simulink model "moving_avg_TB"  (R2024a)
settings: Solver=VariableStepAuto  StartTime=0.0  StopTime=2000  RelTol=1e-3
PreLoadFcn:
  | N = 100;
InitFcn:
  | N = 100;
undefined symbols (not defined in the file or in its folder): Ts
libraries: dspbuff3 x1, simulink x1, dspstat3 x1, dspsrcs4 x1
settings Model: Creator=kschutz  LastModifiedBy=kschutz

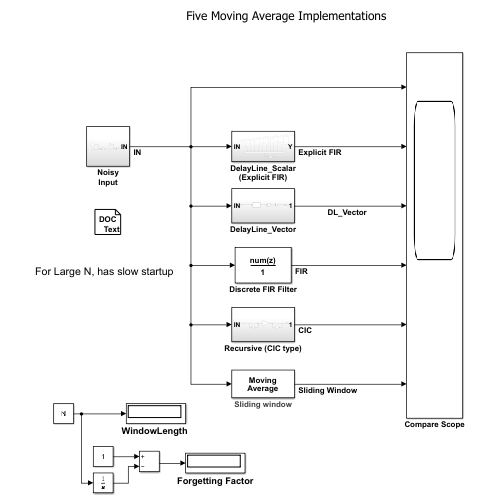
[thumbnail: Simulink's stored preview of the top-level diagram]
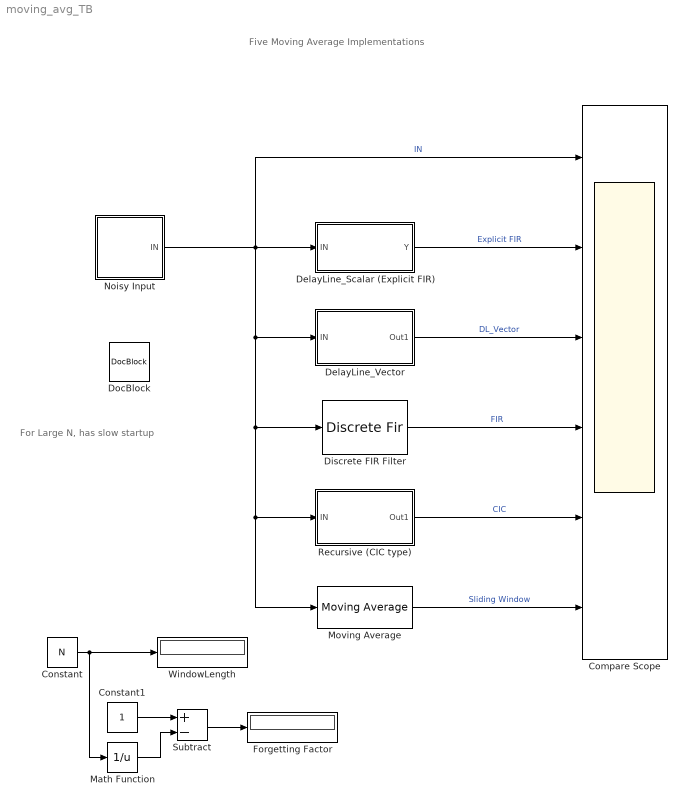
== system moving_avg_TB ==
  note: For Large N, has slow startup
  note: Five Moving Average Implementations
  Compare Scope : Scope  NumInputPorts=6
  Constant : Constant  Value=N
  Constant1 : Constant
  DelayLine_Scalar (Explicit FIR) : Subsystem
  DelayLine_Vector : Subsystem
  Discrete FIR Filter : DiscreteFir  Coefficients=ones(1,N)/N
  DocBlock : simulink/Model-Wide Utilities/DocBlock  DocumentType=Text
      content=|
      | The CIC implementation is the most efficient from a resources perspective,
      | 1 multiplier and two adders. If N is a power of 2, then no multipliers are
      | necessary, just shift logic instead.
  Forgetting Factor : Display
  Math Function : Math  Operator=reciprocal
  Moving Average : dspstat3/Moving Average  Method=Sliding window  ForgettingFactorPort=off  SpecifyWindowLength=on  WindowLength=N  OverlapLength=N-1  AllowArbitraryInputLength=off  ForgettingFactor=1  SimulateUsing=Interpreted execution
      settings: AttributesFormatString=%<Method>
  Noisy Input : Subsystem
  Recursive (CIC type) : Subsystem
  Subtract : Sum  Inputs=+-
  "WindowLength " : Display
  wires:
  Noisy Input/1(IN) -> Compare Scope/1, Moving Average/1, Recursive (CIC type)/1(IN), Discrete FIR Filter/1, DelayLine_Vector/1(IN), DelayLine_Scalar (Explicit FIR)/1(IN)  "IN"
  DelayLine_Scalar (Explicit FIR)/1(Y) -> Compare Scope/2  "Explicit FIR"
  DelayLine_Vector/1(Out1) -> Compare Scope/3  "DL_Vector"
  Discrete FIR Filter/1 -> Compare Scope/4  "FIR"
  Recursive (CIC type)/1(Out1) -> Compare Scope/5  "CIC"
  Moving Average/1 -> Compare Scope/6  "Sliding Window"
  Constant/1 -> "WindowLength "/1, Math Function/1
  Subtract/1 -> Forgetting Factor/1
  Constant1/1 -> Subtract/1
  Math Function/1 -> Subtract/2

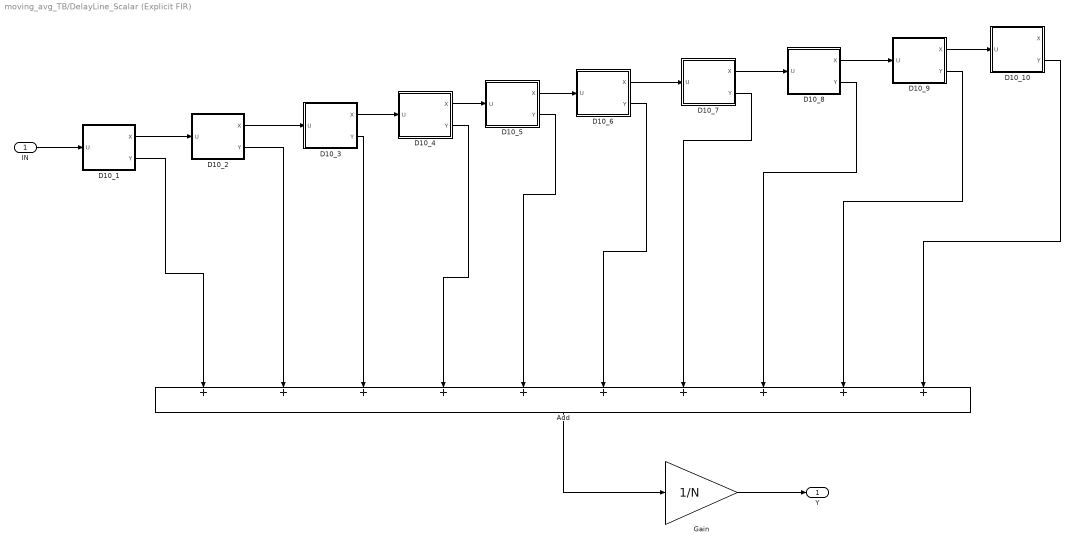
== system moving_avg_TB/DelayLine_Scalar (Explicit FIR) ==
  IN : Inport
  Add : Sum  Inputs=++++++++++
  D10_1 : Subsystem
  D10_10 : Subsystem
  D10_2 : Subsystem
  D10_3 : Subsystem
  D10_4 : Subsystem
  D10_5 : Subsystem
  D10_6 : Subsystem
  D10_7 : Subsystem
  D10_8 : Subsystem
  D10_9 : Subsystem
  Gain : Gain  Gain=1/N
  Y : Outport
  wires:
  IN/1 -> D10_1/1(U)
  D10_1/1(X) -> D10_2/1(U)
  D10_2/1(X) -> D10_3/1(U)
  D10_3/1(X) -> D10_4/1(U)
  D10_4/1(X) -> D10_5/1(U)
  D10_5/1(X) -> D10_6/1(U)
  D10_6/1(X) -> D10_7/1(U)
  D10_7/1(X) -> D10_8/1(U)
  D10_8/1(X) -> D10_9/1(U)
  D10_9/1(X) -> D10_10/1(U)
  D10_1/2(Y) -> Add/1
  Add/1 -> Gain/1
  Gain/1 -> Y/1
  D10_2/2(Y) -> Add/2
  D10_3/2(Y) -> Add/3
  D10_4/2(Y) -> Add/4
  D10_5/2(Y) -> Add/5
  D10_6/2(Y) -> Add/6
  D10_7/2(Y) -> Add/7
  D10_8/2(Y) -> Add/8
  D10_9/2(Y) -> Add/9
  D10_10/2(Y) -> Add/10

== system moving_avg_TB/DelayLine_Vector ==
  IN : Inport
  Delay Line : dspbuff3/Delay Line  siz=N  ic=0  directfeed=on  enable_output=off  hold_output=off  OutputFrames=off
  Gain : Gain  Gain=1/N
  Sum of Elements : Sum  Inputs=+
  Out1 : Outport
  wires:
  Gain/1 -> Out1/1
  Sum of Elements/1 -> Gain/1
  Delay Line/1 -> Sum of Elements/1
  IN/1 -> Delay Line/1

== system moving_avg_TB/Noisy Input ==
  Add : Sum
  Add1 : Sum
  Constant : Constant  SampleTime=1
  Random Source : dspsrcs4/Random Source  SrcType=Gaussian  MinVal=0  MaxVal=1  MeanVal=0  VarVal=.2  RepMode=Specify seed  rawSeed=123  IsInherit=off  SampTime=1  SampFrame=1  OutComplex=Real  DataType=double  SimulateUsing=Interpreted execution
  Step : Step  Time=500  SampleTime=0
  IN : Outport  VectorParamsAs1DForOutWhenUnconnected=off
  wires:
  Constant/1 -> Add1/2
  Random Source/1 -> Add1/1
  Add/1 -> IN/1
  Add1/1 -> Add/2
  Step/1 -> Add/1

== system moving_avg_TB/Recursive (CIC type) ==
  IN : Inport
  Delay : Delay  DelayLength=N
  Delay1 : Delay  DelayLength=1  InputProcessing=Columns as channels (frame based)
  Gain : Gain  Gain=1/N
  Sum : Sum  Inputs=|+-
  Sum1 : Sum  Inputs=|++
  Zero-Order Hold : ZeroOrderHold  Commented=through  SampleTime=Ts
  Out1 : Outport
  wires:
  Sum/1 -> Gain/1
  Sum1/1 -> Out1/1, Delay1/1
  Gain/1 -> Sum1/1
  Delay/1 -> Sum/2
  IN/1 -> Zero-Order Hold/1
  Delay1/1 -> Sum1/2
  Zero-Order Hold/1 -> Delay/1, Sum/1

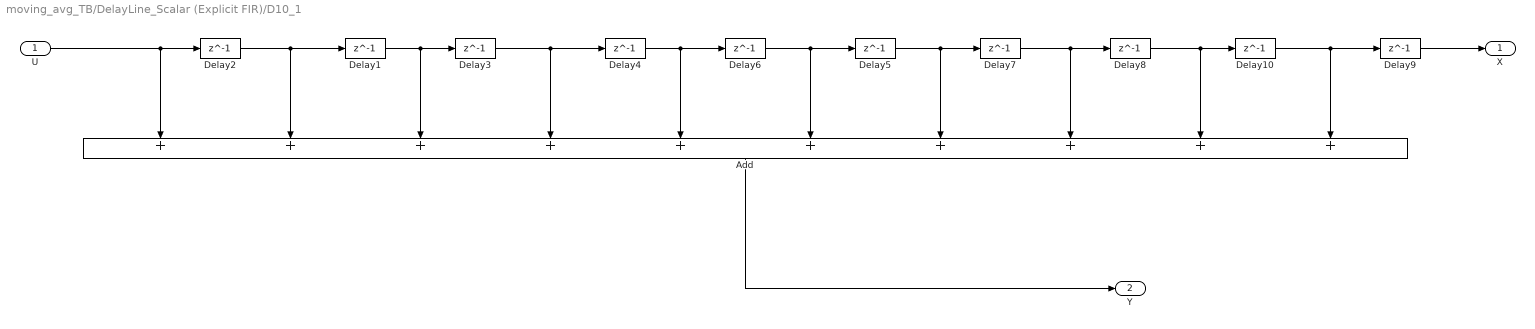
== system moving_avg_TB/DelayLine_Scalar (Explicit FIR)/D10_1 ==
  U : Inport
  Add : Sum  Inputs=++++++++++
  Delay{1..10} (10 alike) : Delay  DelayLength=1  InputProcessing=Columns as channels (frame based)
  X : Outport
  Y : Outport  Port=2
  wires:
  Delay7/1 -> Add/8, Delay8/1
  Delay2/1 -> Add/2, Delay1/1
  Delay3/1 -> Add/4, Delay4/1
  Delay8/1 -> Add/9, Delay10/1
  Delay1/1 -> Delay3/1, Add/3
  Delay6/1 -> Add/6, Delay5/1
  Delay5/1 -> Delay7/1, Add/7
  Delay4/1 -> Add/5, Delay6/1
  U/1 -> Add/1, Delay2/1
  Delay10/1 -> Delay9/1, Add/10
  Add/1 -> Y/1
  Delay9/1 -> X/1

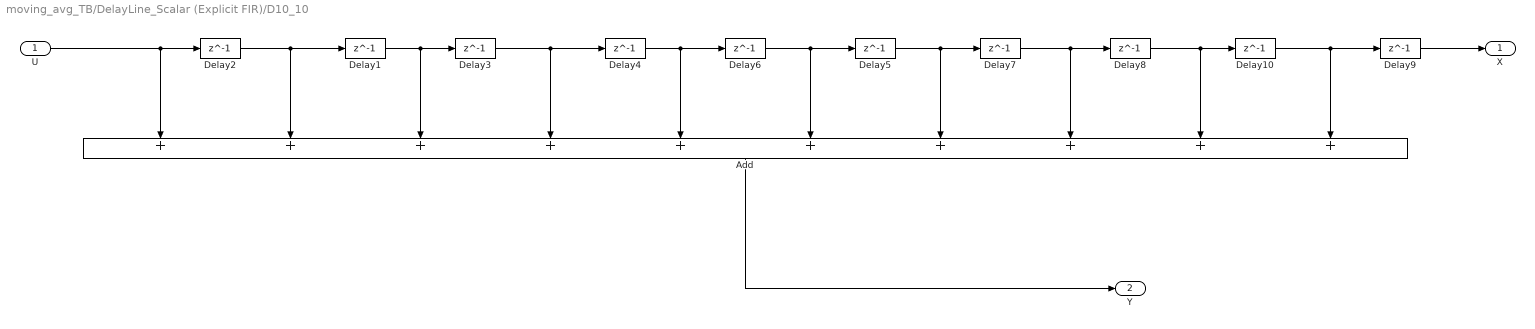
== system moving_avg_TB/DelayLine_Scalar (Explicit FIR)/D10_10 ==
  U : Inport
  Add : Sum  Inputs=++++++++++
  Delay{1..10} (10 alike) : Delay  DelayLength=1  InputProcessing=Columns as channels (frame based)
  X : Outport
  Y : Outport  Port=2
  wires:
  Delay9/1 -> X/1
  Add/1 -> Y/1
  Delay10/1 -> Add/10, Delay9/1
  U/1 -> Delay2/1, Add/1
  Delay4/1 -> Delay6/1, Add/5
  Delay5/1 -> Add/7, Delay7/1
  Delay6/1 -> Delay5/1, Add/6
  Delay1/1 -> Add/3, Delay3/1
  Delay8/1 -> Delay10/1, Add/9
  Delay3/1 -> Delay4/1, Add/4
  Delay2/1 -> Delay1/1, Add/2
  Delay7/1 -> Delay8/1, Add/8

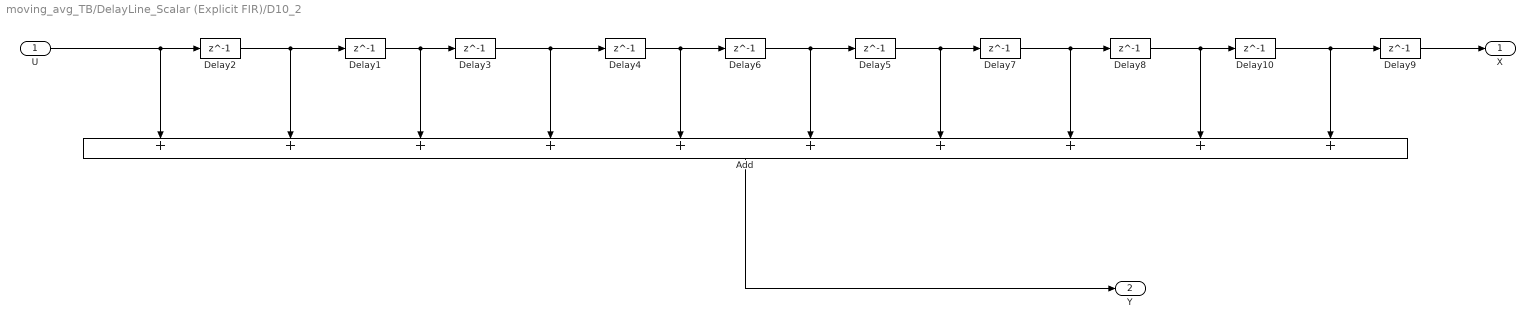
== system moving_avg_TB/DelayLine_Scalar (Explicit FIR)/D10_2 ==
  U : Inport
  Add : Sum  Inputs=++++++++++
  Delay{1..10} (10 alike) : Delay  DelayLength=1  InputProcessing=Columns as channels (frame based)
  X : Outport
  Y : Outport  Port=2
  wires:
  Delay9/1 -> X/1
  Add/1 -> Y/1
  Delay10/1 -> Add/10, Delay9/1
  U/1 -> Delay2/1, Add/1
  Delay4/1 -> Delay6/1, Add/5
  Delay5/1 -> Add/7, Delay7/1
  Delay6/1 -> Delay5/1, Add/6
  Delay1/1 -> Add/3, Delay3/1
  Delay8/1 -> Delay10/1, Add/9
  Delay3/1 -> Delay4/1, Add/4
  Delay2/1 -> Delay1/1, Add/2
  Delay7/1 -> Delay8/1, Add/8

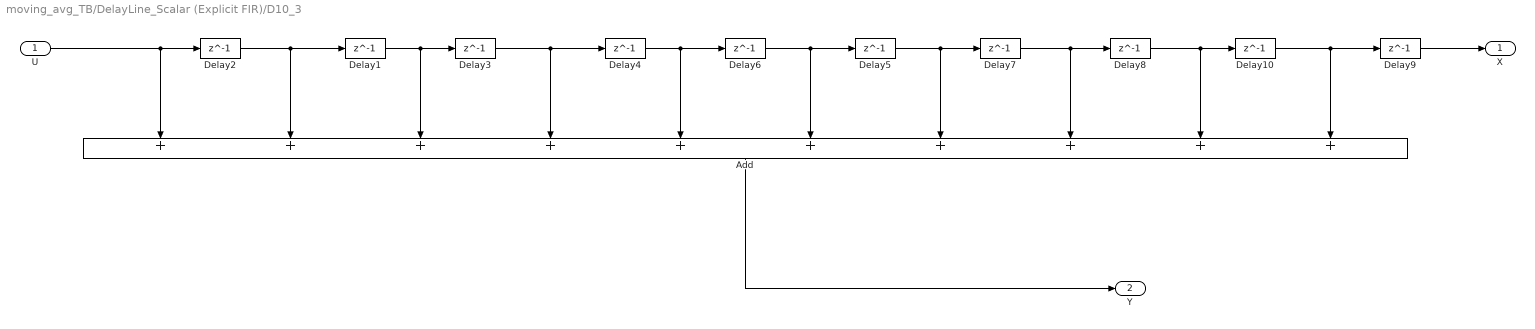
== system moving_avg_TB/DelayLine_Scalar (Explicit FIR)/D10_3 ==
  U : Inport
  Add : Sum  Inputs=++++++++++
  Delay{1..10} (10 alike) : Delay  DelayLength=1  InputProcessing=Columns as channels (frame based)
  X : Outport
  Y : Outport  Port=2
  wires:
  Delay7/1 -> Add/8, Delay8/1
  Delay2/1 -> Add/2, Delay1/1
  Delay3/1 -> Add/4, Delay4/1
  Delay8/1 -> Add/9, Delay10/1
  Delay1/1 -> Delay3/1, Add/3
  Delay6/1 -> Add/6, Delay5/1
  Delay5/1 -> Delay7/1, Add/7
  Delay4/1 -> Add/5, Delay6/1
  U/1 -> Add/1, Delay2/1
  Delay10/1 -> Delay9/1, Add/10
  Add/1 -> Y/1
  Delay9/1 -> X/1

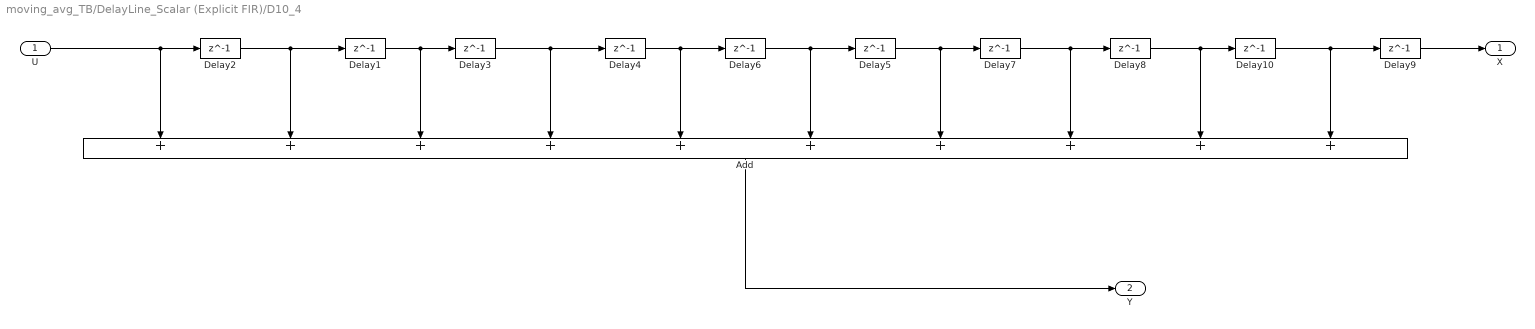
== system moving_avg_TB/DelayLine_Scalar (Explicit FIR)/D10_4 ==
  U : Inport
  Add : Sum  Inputs=++++++++++
  Delay{1..10} (10 alike) : Delay  DelayLength=1  InputProcessing=Columns as channels (frame based)
  X : Outport
  Y : Outport  Port=2
  wires:
  Delay9/1 -> X/1
  Add/1 -> Y/1
  Delay10/1 -> Add/10, Delay9/1
  U/1 -> Delay2/1, Add/1
  Delay4/1 -> Delay6/1, Add/5
  Delay5/1 -> Add/7, Delay7/1
  Delay6/1 -> Delay5/1, Add/6
  Delay1/1 -> Add/3, Delay3/1
  Delay8/1 -> Delay10/1, Add/9
  Delay3/1 -> Delay4/1, Add/4
  Delay2/1 -> Delay1/1, Add/2
  Delay7/1 -> Delay8/1, Add/8

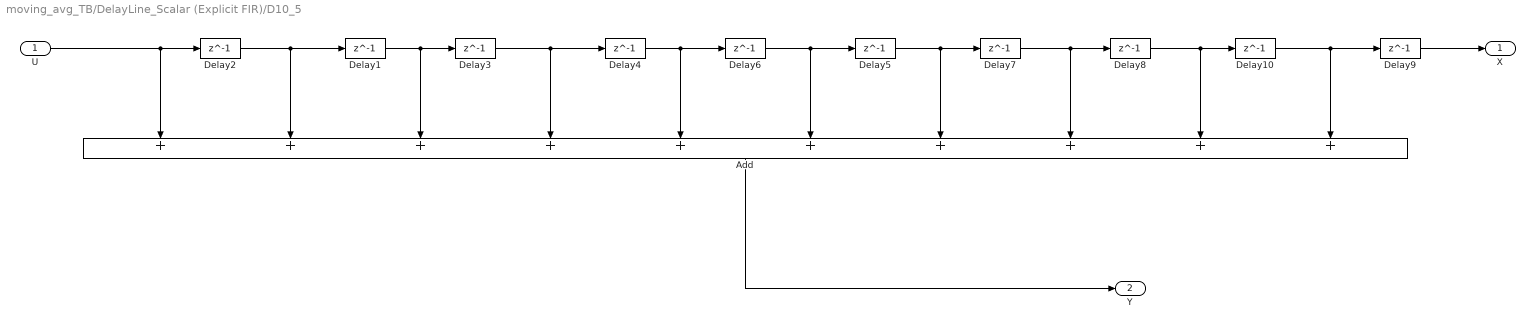
== system moving_avg_TB/DelayLine_Scalar (Explicit FIR)/D10_5 ==
  U : Inport
  Add : Sum  Inputs=++++++++++
  Delay{1..10} (10 alike) : Delay  DelayLength=1  InputProcessing=Columns as channels (frame based)
  X : Outport
  Y : Outport  Port=2
  wires:
  Delay7/1 -> Add/8, Delay8/1
  Delay2/1 -> Add/2, Delay1/1
  Delay3/1 -> Add/4, Delay4/1
  Delay8/1 -> Add/9, Delay10/1
  Delay1/1 -> Delay3/1, Add/3
  Delay6/1 -> Add/6, Delay5/1
  Delay5/1 -> Delay7/1, Add/7
  Delay4/1 -> Add/5, Delay6/1
  U/1 -> Add/1, Delay2/1
  Delay10/1 -> Delay9/1, Add/10
  Add/1 -> Y/1
  Delay9/1 -> X/1

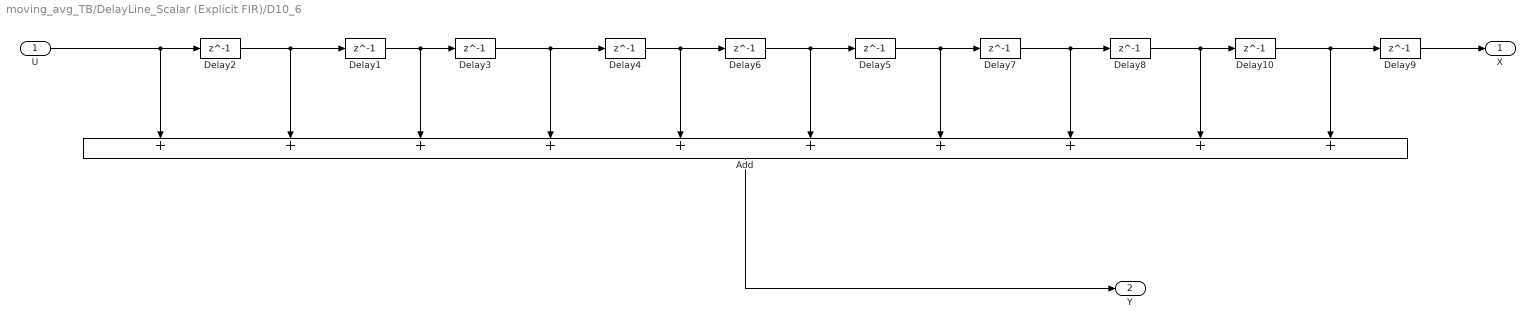
== system moving_avg_TB/DelayLine_Scalar (Explicit FIR)/D10_6 ==
  U : Inport
  Add : Sum  Inputs=++++++++++
  Delay{1..10} (10 alike) : Delay  DelayLength=1  InputProcessing=Columns as channels (frame based)
  X : Outport
  Y : Outport  Port=2
  wires:
  Delay9/1 -> X/1
  Add/1 -> Y/1
  Delay10/1 -> Add/10, Delay9/1
  U/1 -> Delay2/1, Add/1
  Delay4/1 -> Delay6/1, Add/5
  Delay5/1 -> Add/7, Delay7/1
  Delay6/1 -> Delay5/1, Add/6
  Delay1/1 -> Add/3, Delay3/1
  Delay8/1 -> Delay10/1, Add/9
  Delay3/1 -> Delay4/1, Add/4
  Delay2/1 -> Delay1/1, Add/2
  Delay7/1 -> Delay8/1, Add/8

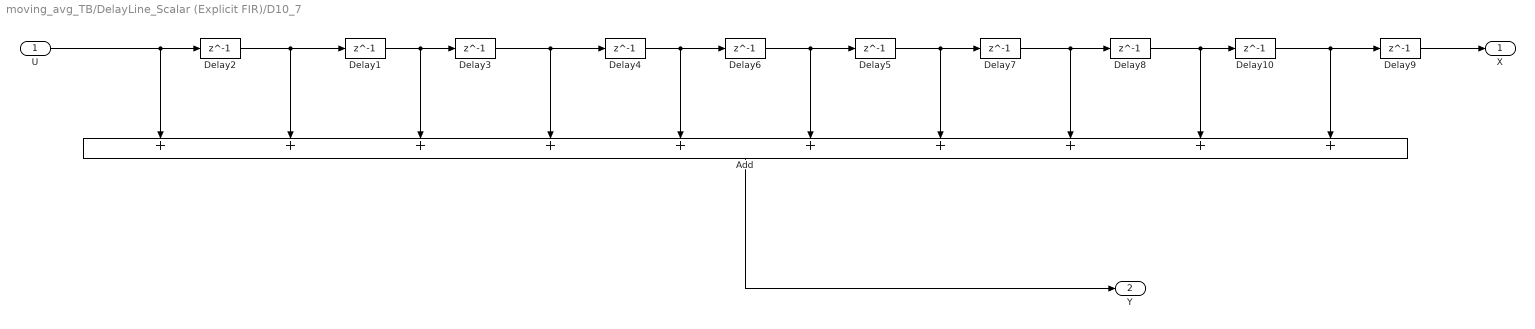
== system moving_avg_TB/DelayLine_Scalar (Explicit FIR)/D10_7 ==
  U : Inport
  Add : Sum  Inputs=++++++++++
  Delay{1..10} (10 alike) : Delay  DelayLength=1  InputProcessing=Columns as channels (frame based)
  X : Outport
  Y : Outport  Port=2
  wires:
  Delay7/1 -> Add/8, Delay8/1
  Delay2/1 -> Add/2, Delay1/1
  Delay3/1 -> Add/4, Delay4/1
  Delay8/1 -> Add/9, Delay10/1
  Delay1/1 -> Delay3/1, Add/3
  Delay6/1 -> Add/6, Delay5/1
  Delay5/1 -> Delay7/1, Add/7
  Delay4/1 -> Add/5, Delay6/1
  U/1 -> Add/1, Delay2/1
  Delay10/1 -> Delay9/1, Add/10
  Add/1 -> Y/1
  Delay9/1 -> X/1

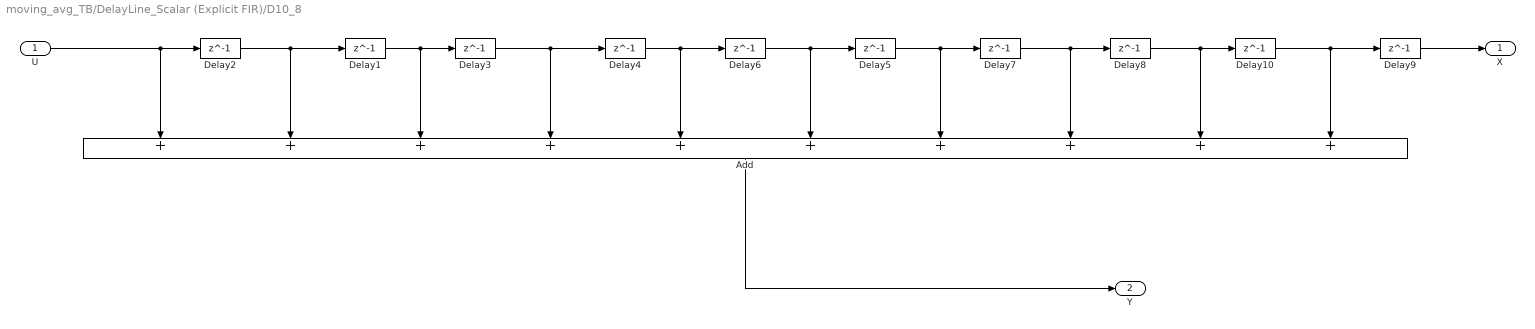
== system moving_avg_TB/DelayLine_Scalar (Explicit FIR)/D10_8 ==
  U : Inport
  Add : Sum  Inputs=++++++++++
  Delay{1..10} (10 alike) : Delay  DelayLength=1  InputProcessing=Columns as channels (frame based)
  X : Outport
  Y : Outport  Port=2
  wires:
  Delay9/1 -> X/1
  Add/1 -> Y/1
  Delay10/1 -> Add/10, Delay9/1
  U/1 -> Delay2/1, Add/1
  Delay4/1 -> Delay6/1, Add/5
  Delay5/1 -> Add/7, Delay7/1
  Delay6/1 -> Delay5/1, Add/6
  Delay1/1 -> Add/3, Delay3/1
  Delay8/1 -> Delay10/1, Add/9
  Delay3/1 -> Delay4/1, Add/4
  Delay2/1 -> Delay1/1, Add/2
  Delay7/1 -> Delay8/1, Add/8

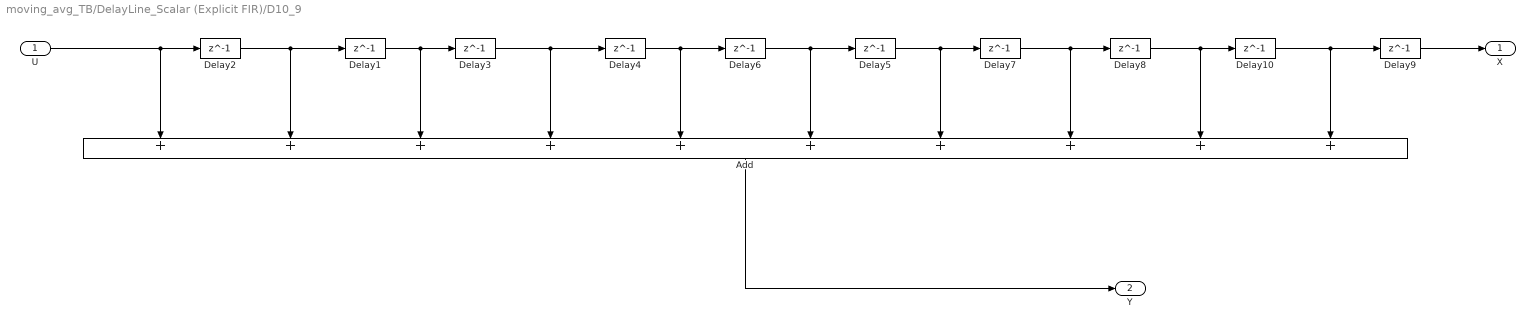
== system moving_avg_TB/DelayLine_Scalar (Explicit FIR)/D10_9 ==
  U : Inport
  Add : Sum  Inputs=++++++++++
  Delay{1..10} (10 alike) : Delay  DelayLength=1  InputProcessing=Columns as channels (frame based)
  X : Outport
  Y : Outport  Port=2
  wires:
  Delay7/1 -> Add/8, Delay8/1
  Delay2/1 -> Add/2, Delay1/1
  Delay3/1 -> Add/4, Delay4/1
  Delay8/1 -> Add/9, Delay10/1
  Delay1/1 -> Delay3/1, Add/3
  Delay6/1 -> Add/6, Delay5/1
  Delay5/1 -> Delay7/1, Add/7
  Delay4/1 -> Add/5, Delay6/1
  U/1 -> Add/1, Delay2/1
  Delay10/1 -> Delay9/1, Add/10
  Add/1 -> Y/1
  Delay9/1 -> X/1
